simulink model "PID_P_S_I"  (R2023b)
settings: Solver=VariableStepAuto  StartTime=0.0  StopTime=10.0  RelTol=1e-3
libraries: simulink x3
settings Model: Creator=ascom  LastModifiedBy=ascom

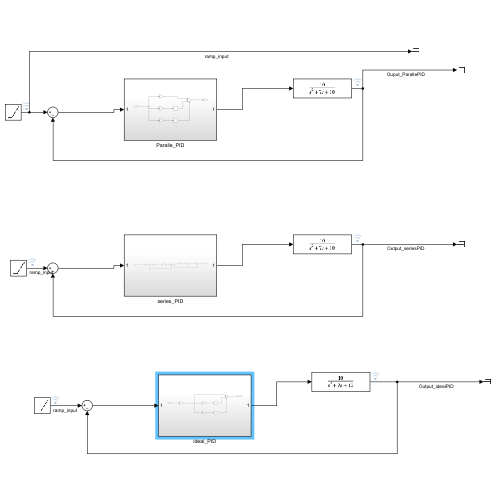
[thumbnail: Simulink's stored preview of the top-level diagram]
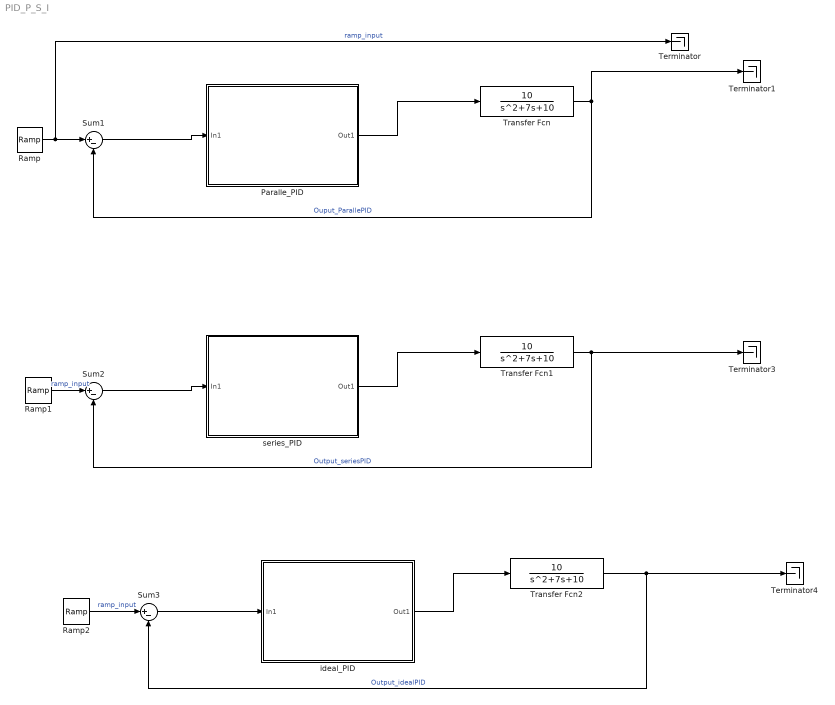
== system PID_P_S_I ==
  Paralle_PID : Subsystem
  Ramp : simulink/Sources/Ramp  slope=1  start=0  InitialOutput=0
  Ramp1 : simulink/Sources/Ramp  slope=1  start=0  InitialOutput=0
  Ramp2 : simulink/Sources/Ramp  slope=1  start=0  InitialOutput=0
  Sum1 : Sum  Inputs=|+-
  Sum2 : Sum  Inputs=|+-
  Sum3 : Sum  Inputs=|+-
  Terminator{,1,3..4} (4 alike) : Terminator
  Transfer Fcn : TransferFcn  Numerator=[10]  Denominator=[1 7 10]
  Transfer Fcn1 : TransferFcn  Numerator=[10]  Denominator=[1 7 10]
  Transfer Fcn2 : TransferFcn  Numerator=[10]  Denominator=[1 7 10]
  ideal_PID : Subsystem
  series_PID : Subsystem
  wires:
  Transfer Fcn/1 -> Terminator1/1, Sum1/2  "Ouput_ParallePID"
  Ramp/1 -> Terminator/1, Sum1/1  "ramp_input"
  Sum1/1 -> Paralle_PID/1(In1)
  Paralle_PID/1(Out1) -> Transfer Fcn/1
  series_PID/1(Out1) -> Transfer Fcn1/1
  Ramp1/1 -> Sum2/1  "ramp_input"
  Sum2/1 -> series_PID/1(In1)
  Transfer Fcn1/1 -> Terminator3/1, Sum2/2  "Output_seriesPID"
  ideal_PID/1(Out1) -> Transfer Fcn2/1
  Ramp2/1 -> Sum3/1  "ramp_input"
  Sum3/1 -> ideal_PID/1(In1)
  Transfer Fcn2/1 -> Terminator4/1, Sum3/2  "Output_idealPID"

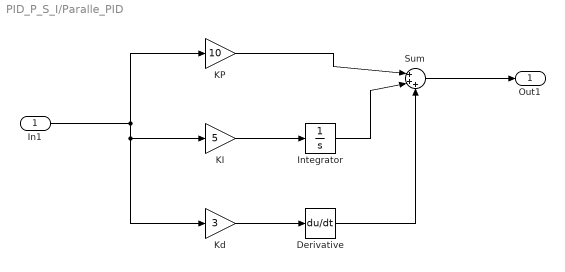
== system PID_P_S_I/Paralle_PID ==
  In1 : Inport
  Derivative : Derivative
  Integrator : Integrator
  KI : Gain  Gain=5
  KP : Gain  Gain=10
  Kd : Gain  Gain=3
  Sum : Sum  Inputs=|+++
  Out1 : Outport
  wires:
  Kd/1 -> Derivative/1
  Derivative/1 -> Sum/3
  KI/1 -> Integrator/1
  In1/1 -> Kd/1, KI/1, KP/1
  Integrator/1 -> Sum/2
  KP/1 -> Sum/1
  Sum/1 -> Out1/1

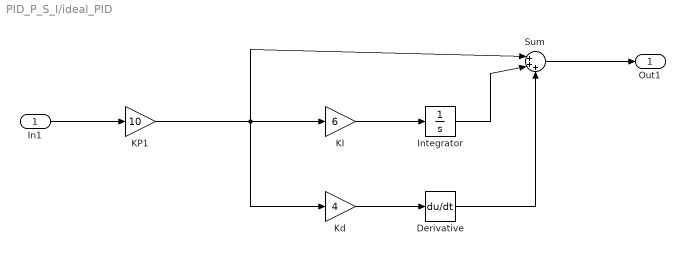
== system PID_P_S_I/ideal_PID ==
  In1 : Inport
  Derivative : Derivative
  Integrator : Integrator
  KI : Gain  Gain=6
  KP1 : Gain  Gain=10
  Kd : Gain  Gain=4
  Sum : Sum  Inputs=|+++
  Out1 : Outport
  wires:
  Kd/1 -> Derivative/1
  Derivative/1 -> Sum/3
  KI/1 -> Integrator/1
  Integrator/1 -> Sum/2
  In1/1 -> KP1/1
  Sum/1 -> Out1/1
  KP1/1 -> Sum/1, Kd/1, KI/1

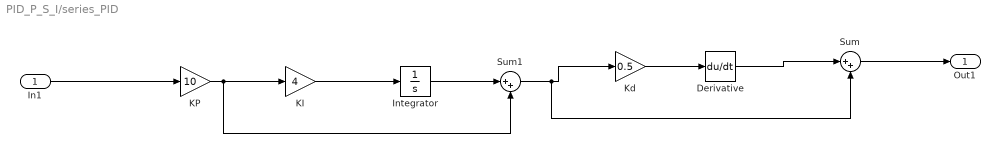
== system PID_P_S_I/series_PID ==
  In1 : Inport
  Derivative : Derivative
  Integrator : Integrator
  KI : Gain  Gain=4
  KP : Gain  Gain=10
  Kd : Gain  Gain=0.5
  Sum : Sum  Inputs=|++
  Sum1 : Sum  Inputs=|++
  Out1 : Outport
  wires:
  Kd/1 -> Derivative/1
  KI/1 -> Integrator/1
  In1/1 -> KP/1
  Sum/1 -> Out1/1
  Integrator/1 -> Sum1/1
  KP/1 -> Sum1/2, KI/1
  Sum1/1 -> Sum/2, Kd/1
  Derivative/1 -> Sum/1
